simulink model "LgrstCloseRStateCtrl"  (R2018b)
settings: Solver=FixedStepDiscrete  StartTime=0.0  StopTime=10.0  FixedStep=0.01  RelTol=1e-3
libraries: StateCtrlLib x1
settings Model: Creator=sn2xws  LastModifiedBy=sn2xws
settings DataIOCC: SaveFormat=StructureWithTime
settings OptimizationCC: DefaultParameterBehavior=Inlined  EnhancedBackFolding=on  PassReuseOutputArgsAs=Individual arguments  ZeroExternalMemoryAtStartup=off  ZeroInternalMemoryAtStartup=off  OptimizeBlockOrder=speed  DifferentSizesBufferReuse=on  OptimizationCustomize=off
settings DebuggingCC: ParameterTunabilityLossMsg=error
settings ModelReferenceCC: ModelReferenceNumInstancesAllowed=Single
settings SFSimCC: MATLABDynamicMemAlloc=off
settings RTWCC: SystemTargetFile=autosar.tlc  GenCodeOnly=on  TemplateMakefile=ert_default_tmf  Description=AUTOSAR  GenerateReport=on  IncludeHyperlinkInReport=on  LaunchReport=on  GenerateTraceInfo=on  GenerateTraceReport=on  GenerateTraceReportSl=on  GenerateTraceReportSf=on  GenerateTraceReportEml=on
settings CodeAppCC: ForceParamTrailComments=on  IgnoreCustomStorageClasses=off  OperatorAnnotations=on  SimulinkDataObjDesc=on  SFDataObjDesc=on  InsertBlockDesc=on
settings STFCustomTargetCC: TargetLangStandard=C99 (ISO)  MultiwordLength=256  ParMdlRefBuildCompliant=on  CompOptLevelCompliant=on  IncludeMdlTerminateFcn=off  CombineOutputUpdateFcns=on  SuppressErrorStatus=on  ERTCustomFileBanners=on  SupportNonFinite=off  SupportComplex=off  SupportContinuousTime=off  SupportNonInlinedSFcns=off  RemoveResetFunc=on  MATLABClassNameForMDSCustomization=Simulink.SoftwareTarget.ERTCustomization  AutosarCompliant=on  UseToolchainInfoCompliant=on  LookupTableObjectStructAxisOrder=2,1,3,4,...  LUTObjectStructOrderEvenSpacing=Size,Table,Breakpoints  SystemTargetFile=autosar.tlc
settings ERTTargetCC: TargetLangStandard=C99 (ISO)  ConcurrentExecutionCompliant=off  IncludeMdlTerminateFcn=off  SuppressErrorStatus=on  SupportNonFinite=off  SupportComplex=off  ModelStepFunctionPrototypeControlCompliant=off  CPPClassGenCompliant=off  AutosarCompliant=on  LookupTableObjectStructAxisOrder=2,1,3,4,...  LUTObjectStructOrderEvenSpacing=Size,Table,Breakpoints  InlinedParameterPlacement=NonHierarchical  ERTCustomFileTemplate=example_file_process.tlc

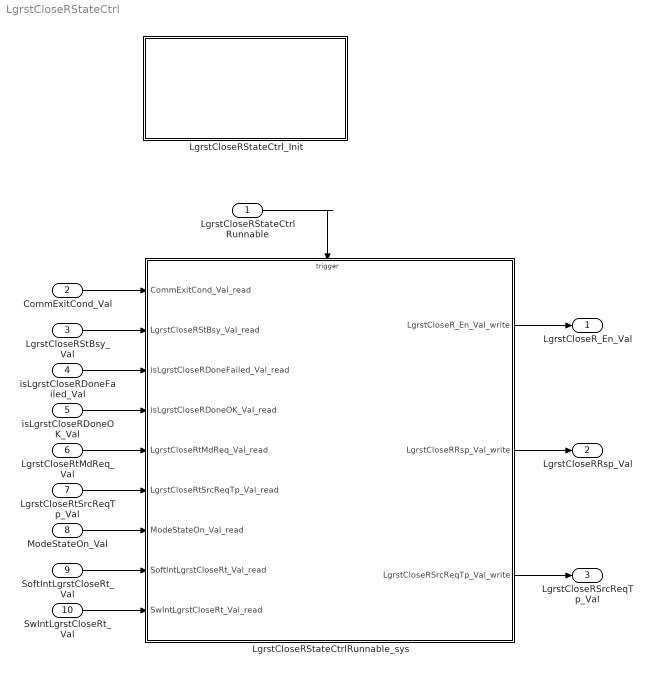
== system LgrstCloseRStateCtrl ==
  LgrstCloseRStateCtrlRunnable : Inport  SampleTime=0.01  OutputFunctionCall=on
  CommExitCond_Val : Inport  Port=2  OutDataTypeStr=boolean  PortDimensions=1
  LgrstCloseRStBsy_Val : Inport  Port=3  OutDataTypeStr=boolean  PortDimensions=1
  isLgrstCloseRDoneFailed_Val : Inport  Port=4  OutDataTypeStr=boolean  PortDimensions=1
  isLgrstCloseRDoneOK_Val : Inport  Port=5  OutDataTypeStr=boolean  PortDimensions=1
  LgrstCloseRtMdReq_Val : Inport  Port=6  OutDataTypeStr=boolean  PortDimensions=1
  LgrstCloseRtSrcReqTp_Val : Inport  Port=7  OutDataTypeStr=Enum: SrcReqTp1  PortDimensions=1
  ModeStateOn_Val : Inport  Port=8  OutDataTypeStr=boolean  PortDimensions=1
  SoftIntLgrstCloseRt_Val : Inport  Port=9  OutDataTypeStr=IntEnable  PortDimensions=1
  SwIntLgrstCloseRt_Val : Inport  Port=10  OutDataTypeStr=IntEnable  PortDimensions=1
  LgrstCloseRStateCtrlRunnable_sys : Subsystem
  LgrstCloseRStateCtrl_Init : Subsystem
  LgrstCloseR_En_Val : Outport  OutDataTypeStr=boolean  PortDimensions=1
  LgrstCloseRRsp_Val : Outport  Port=2  OutDataTypeStr=Enum: MdRspLocal1  PortDimensions=1
  LgrstCloseRSrcReqTp_Val : Outport  Port=3  OutDataTypeStr=Enum: SrcReqTp1  PortDimensions=1
  wires:
  CommExitCond_Val/1 -> LgrstCloseRStateCtrlRunnable_sys/1(CommExitCond_Val_read)
  LgrstCloseRStBsy_Val/1 -> LgrstCloseRStateCtrlRunnable_sys/2(LgrstCloseRStBsy_Val_read)
  isLgrstCloseRDoneFailed_Val/1 -> LgrstCloseRStateCtrlRunnable_sys/3(isLgrstCloseRDoneFailed_Val_read)
  isLgrstCloseRDoneOK_Val/1 -> LgrstCloseRStateCtrlRunnable_sys/4(isLgrstCloseRDoneOK_Val_read)
  LgrstCloseRtMdReq_Val/1 -> LgrstCloseRStateCtrlRunnable_sys/5(LgrstCloseRtMdReq_Val_read)
  LgrstCloseRtSrcReqTp_Val/1 -> LgrstCloseRStateCtrlRunnable_sys/6(LgrstCloseRtSrcReqTp_Val_read)
  ModeStateOn_Val/1 -> LgrstCloseRStateCtrlRunnable_sys/7(ModeStateOn_Val_read)
  SoftIntLgrstCloseRt_Val/1 -> LgrstCloseRStateCtrlRunnable_sys/8(SoftIntLgrstCloseRt_Val_read)
  SwIntLgrstCloseRt_Val/1 -> LgrstCloseRStateCtrlRunnable_sys/9(SwIntLgrstCloseRt_Val_read)
  LgrstCloseRStateCtrlRunnable_sys/1(LgrstCloseR_En_Val_write) -> LgrstCloseR_En_Val/1
  LgrstCloseRStateCtrlRunnable_sys/2(LgrstCloseRRsp_Val_write) -> LgrstCloseRRsp_Val/1
  LgrstCloseRStateCtrlRunnable_sys/3(LgrstCloseRSrcReqTp_Val_write) -> LgrstCloseRSrcReqTp_Val/1
  LgrstCloseRStateCtrlRunnable/1 -> LgrstCloseRStateCtrlRunnable_sys/Trigger

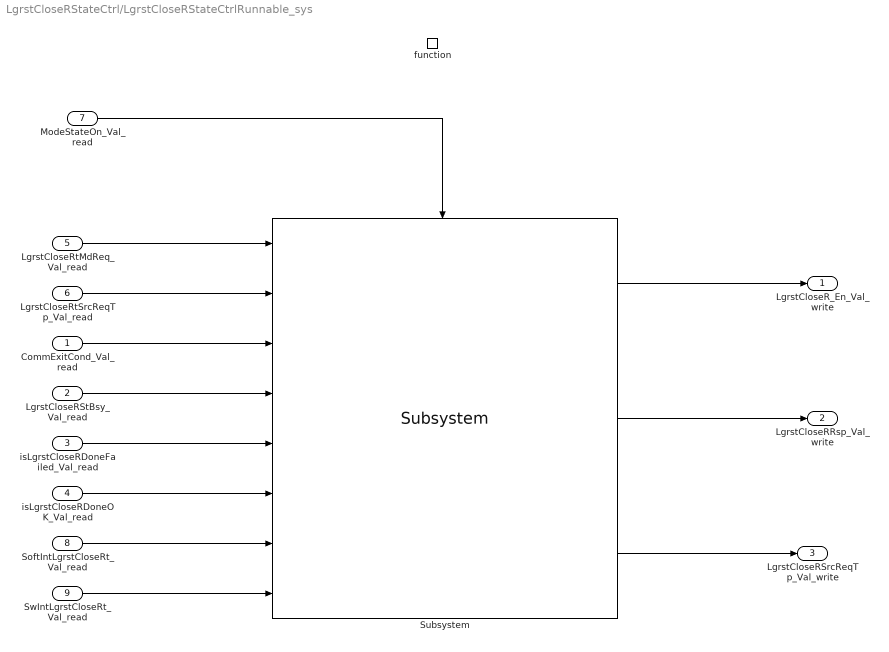
== system LgrstCloseRStateCtrl/LgrstCloseRStateCtrlRunnable_sys ==
  CommExitCond_Val_read : Inport
  LgrstCloseRStBsy_Val_read : Inport  Port=2
  isLgrstCloseRDoneFailed_Val_read : Inport  Port=3
  isLgrstCloseRDoneOK_Val_read : Inport  Port=4
  LgrstCloseRtMdReq_Val_read : Inport  Port=5
  LgrstCloseRtSrcReqTp_Val_read : Inport  Port=6
  ModeStateOn_Val_read : Inport  Port=7
  SoftIntLgrstCloseRt_Val_read : Inport  Port=8
  SwIntLgrstCloseRt_Val_read : Inport  Port=9
  function : TriggerPort  TriggerType=function-call  VariantControl=(inherit)  SampleTimeType=periodic  SampleTime=-1
  Subsystem : StateCtrlLib/Subsystem  SystemSampleTime=-1
  LgrstCloseR_En_Val_write : Outport
      settings: EnsureOutportIsVirtual=on
  LgrstCloseRRsp_Val_write : Outport  Port=2
      settings: EnsureOutportIsVirtual=on
  LgrstCloseRSrcReqTp_Val_write : Outport  Port=3
      settings: EnsureOutportIsVirtual=on
  wires:
  Subsystem/2 -> LgrstCloseRRsp_Val_write/1
  Subsystem/1 -> LgrstCloseR_En_Val_write/1
  Subsystem/3 -> LgrstCloseRSrcReqTp_Val_write/1
  ModeStateOn_Val_read/1 -> Subsystem/Enable
  LgrstCloseRtMdReq_Val_read/1 -> Subsystem/1
  CommExitCond_Val_read/1 -> Subsystem/3
  LgrstCloseRtSrcReqTp_Val_read/1 -> Subsystem/2
  LgrstCloseRStBsy_Val_read/1 -> Subsystem/4
  isLgrstCloseRDoneFailed_Val_read/1 -> Subsystem/5
  SoftIntLgrstCloseRt_Val_read/1 -> Subsystem/7
  isLgrstCloseRDoneOK_Val_read/1 -> Subsystem/6
  SwIntLgrstCloseRt_Val_read/1 -> Subsystem/8

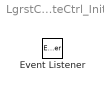
== system LgrstCloseRStateCtrl/LgrstCloseRStateCtrl_Init ==
  Event Listener : EventListener  EventName=reset
